simulink model "quadrotor_Euler"  (R2022b)
settings: Solver=VariableStepAuto  StartTime=0.0  StopTime=10.0  RelTol=1e-3
libraries: slpidlib x4
settings Model: SnapshotBufferSize=20  SnapshotInterval=20  Creator=user  LastModifiedBy=user

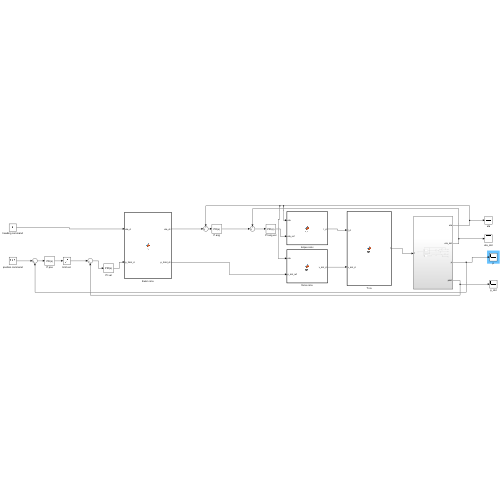
[thumbnail: Simulink's stored preview of the top-level diagram]
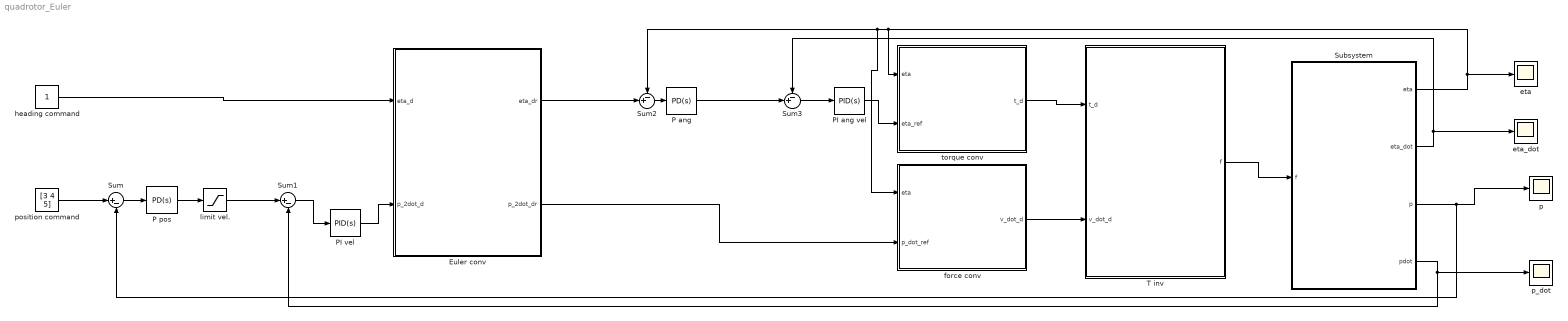
== system quadrotor_Euler ==
  Euler conv : MATLAB Function  TreatAsAtomicUnit=on
  P ang : slpidlib/PID Controller  Controller=PD  Form=Parallel  TimeDomain=Continuous-time  UseExternalTs=off  SampleTime=-1  IntegratorMethod=Forward Euler  FilterMethod=Forward Euler  ControllerParametersSource=internal  P=20  I=1  UseKiTs=off  D=0.2  N=100  UseFilter=on  TunerSelectOption=Transfer Function Based (PID Tuner App)  InitialConditionSource=internal  InitialConditionForIntegrator=0  InitialConditionForFilter=0  DifferentiatorICPrevScaledInput=0  ExternalReset=none  TrackingMode=off  Kt=1  LimitOutput=off  SatLimitsSource=internal  UpperSaturationLimit=inf  LowerSaturationLimit=-inf  LinearizeAsGain=on  AntiWindupMode=none  Kb=1  LimitIntegrator=off  UpperIntegratorSaturationLimit=inf  LowerIntegratorSaturationLimit=-inf  POutMin=[]  POutMax=[]  IOutMin=[]  IOutMax=[]  DOutMin=[]  DOutMax=[]  NOutMin=[]  NOutMax=[]  SumOutMin=[]  SumOutMax=[]  SaturationOutMin=[]  SaturationOutMax=[]  PParamMin=[]  PParamMax=[]  IParamMin=[]  IParamMax=[]  DParamMin=[]  DParamMax=[]  NParamMin=[]  NParamMax=[]  KbParamMin=[]  KbParamMax=[]  KtParamMin=[]  KtParamMax=[]  KbOutMin=[]  KbOutMax=[]  KtOutMin=[]  KtOutMax=[]  IntegratorOutMin=[]  IntegratorOutMax=[]  FilterOutMin=[]  FilterOutMax=[]  SumI1OutMin=[]  SumI1OutMax=[]  SumI2OutMin=[]  SumI2OutMax=[]  SumI3OutMin=[]  SumI3OutMax=[]  SumI4OutMin=[]  SumI4OutMax=[]  SumDOutMin=[]  SumDOutMax=[]  DifferentiatorOutMin=[]  DifferentiatorOutMax=[]  FilterDiffOutCoefMin=[]  FilterDiffOutCoefMax=[]  ReciprocalOutMin=[]  ReciprocalOutMax=[]  SumDenOutMin=[]  SumDenOutMax=[]  SumNumOutMin=[]  SumNumOutMax=[]  DivideOutMin=[]  DivideOutMax=[]  UdiffTsProdOutMin=[]  UdiffTsProdOutMax=[]  NTsProdOutMin=[]  NTsProdOutMax=[]  UintegralTsProdOutMin=[]  UintegralTsProdOutMax=[]  UngainTsProdOutMin=[]  UngainTsProdOutMax=[]  ClampingZeroOutDataTypeStr=Inherit: Inherit via back propagation  ClampingZeroOutMin=[]  ClampingZeroOutMax=[]  FilterDenConstantOutDataTypeStr=Inherit: Inherit via back propagation  FilterDenConstantOutMin=[]  FilterDenConstantOutMax=[]  PCopyOutDataTypeStr=Inherit: Inherit via back propagation  PCopyOutMin=[]  PCopyOutMax=[]  NCopyOutDataTypeStr=Inherit: Inherit via back propagation  NCopyOutMin=[]  NCopyOutMax=[]  IntegratorContinuousStateAttributes=''  IntegratorStateMustResolveToSignalObject=off  IntegratorRTWStateStorageClass=Auto  FilterContinuousStateAttributes=''  FilterStateMustResolveToSignalObject=off  FilterRTWStateStorageClass=Auto  ParallelPVariant=InternalParameters  IdealPVariant=Disabled  IVariant=Disabled  DVariant=InternalParameters  IntegratorVariant=Disabled  SatVariant=Disabled  AWVariant=Disabled  PCopyVariant=Disabled  TRVariant=Disabled  FdbkBlocksVariant=Forward  IdealPFdbkVariant=Disabled  SatFdbkVariant=Disabled  DerivativeFilterVariant=ContFilter  NVariant=InternalParameters  NCopyVariant=Disabled  FilterICVariant=InternalICsFilter  IntegratorICVariant=Disabled  ExternalResetVariant=Disabled  TRSumVariant=Passthrough  SumFdbkVariant=Disabled  SumVariant=Sum_PD  TsampFilterVariant=InternalTs  TsampNgainVariant=Passthrough  TsampIntegralVariant=Disabled_SignalSpec  ExternalSaturationOutDataTypeStr=Inherit: Same as second input
  P pos : slpidlib/PID Controller  Controller=PD  Form=Parallel  TimeDomain=Continuous-time  UseExternalTs=off  SampleTime=-1  IntegratorMethod=Forward Euler  FilterMethod=Forward Euler  ControllerParametersSource=internal  P=5  I=1  UseKiTs=off  D=0.8  N=100  UseFilter=on  TunerSelectOption=Transfer Function Based (PID Tuner App)  InitialConditionSource=internal  InitialConditionForIntegrator=0  InitialConditionForFilter=0  DifferentiatorICPrevScaledInput=0  ExternalReset=none  TrackingMode=off  Kt=1  LimitOutput=off  SatLimitsSource=internal  UpperSaturationLimit=inf  LowerSaturationLimit=-inf  LinearizeAsGain=on  AntiWindupMode=none  Kb=1  LimitIntegrator=off  UpperIntegratorSaturationLimit=inf  LowerIntegratorSaturationLimit=-inf  POutMin=[]  POutMax=[]  IOutMin=[]  IOutMax=[]  DOutMin=[]  DOutMax=[]  NOutMin=[]  NOutMax=[]  SumOutMin=[]  SumOutMax=[]  SaturationOutMin=[]  SaturationOutMax=[]  PParamMin=[]  PParamMax=[]  IParamMin=[]  IParamMax=[]  DParamMin=[]  DParamMax=[]  NParamMin=[]  NParamMax=[]  KbParamMin=[]  KbParamMax=[]  KtParamMin=[]  KtParamMax=[]  KbOutMin=[]  KbOutMax=[]  KtOutMin=[]  KtOutMax=[]  IntegratorOutMin=[]  IntegratorOutMax=[]  FilterOutMin=[]  FilterOutMax=[]  SumI1OutMin=[]  SumI1OutMax=[]  SumI2OutMin=[]  SumI2OutMax=[]  SumI3OutMin=[]  SumI3OutMax=[]  SumI4OutMin=[]  SumI4OutMax=[]  SumDOutMin=[]  SumDOutMax=[]  DifferentiatorOutMin=[]  DifferentiatorOutMax=[]  FilterDiffOutCoefMin=[]  FilterDiffOutCoefMax=[]  ReciprocalOutMin=[]  ReciprocalOutMax=[]  SumDenOutMin=[]  SumDenOutMax=[]  SumNumOutMin=[]  SumNumOutMax=[]  DivideOutMin=[]  DivideOutMax=[]  UdiffTsProdOutMin=[]  UdiffTsProdOutMax=[]  NTsProdOutMin=[]  NTsProdOutMax=[]  UintegralTsProdOutMin=[]  UintegralTsProdOutMax=[]  UngainTsProdOutMin=[]  UngainTsProdOutMax=[]  ClampingZeroOutDataTypeStr=Inherit: Inherit via back propagation  ClampingZeroOutMin=[]  ClampingZeroOutMax=[]  FilterDenConstantOutDataTypeStr=Inherit: Inherit via back propagation  FilterDenConstantOutMin=[]  FilterDenConstantOutMax=[]  PCopyOutDataTypeStr=Inherit: Inherit via back propagation  PCopyOutMin=[]  PCopyOutMax=[]  NCopyOutDataTypeStr=Inherit: Inherit via back propagation  NCopyOutMin=[]  NCopyOutMax=[]  IntegratorContinuousStateAttributes=''  IntegratorStateMustResolveToSignalObject=off  IntegratorRTWStateStorageClass=Auto  FilterContinuousStateAttributes=''  FilterStateMustResolveToSignalObject=off  FilterRTWStateStorageClass=Auto  ParallelPVariant=InternalParameters  IdealPVariant=Disabled  IVariant=Disabled  DVariant=InternalParameters  IntegratorVariant=Disabled  SatVariant=Disabled  AWVariant=Disabled  PCopyVariant=Disabled  TRVariant=Disabled  FdbkBlocksVariant=Forward  IdealPFdbkVariant=Disabled  SatFdbkVariant=Disabled  DerivativeFilterVariant=ContFilter  NVariant=InternalParameters  NCopyVariant=Disabled  FilterICVariant=InternalICsFilter  IntegratorICVariant=Disabled  ExternalResetVariant=Disabled  TRSumVariant=Passthrough  SumFdbkVariant=Disabled  SumVariant=Sum_PD  TsampFilterVariant=InternalTs  TsampNgainVariant=Passthrough  TsampIntegralVariant=Disabled_SignalSpec  ExternalSaturationOutDataTypeStr=Inherit: Same as second input
  PI ang vel : slpidlib/PID Controller  Controller=PID  Form=Parallel  TimeDomain=Continuous-time  UseExternalTs=off  SampleTime=-1  IntegratorMethod=Forward Euler  FilterMethod=Forward Euler  ControllerParametersSource=internal  P=25  I=0.0  UseKiTs=off  D=0  N=100  UseFilter=on  TunerSelectOption=Transfer Function Based (PID Tuner App)  InitialConditionSource=internal  InitialConditionForIntegrator=0  InitialConditionForFilter=0  DifferentiatorICPrevScaledInput=0  ExternalReset=none  TrackingMode=off  Kt=1  LimitOutput=off  SatLimitsSource=internal  UpperSaturationLimit=inf  LowerSaturationLimit=-inf  LinearizeAsGain=on  AntiWindupMode=none  Kb=1  LimitIntegrator=off  UpperIntegratorSaturationLimit=inf  LowerIntegratorSaturationLimit=-inf  POutMin=[]  POutMax=[]  IOutMin=[]  IOutMax=[]  DOutMin=[]  DOutMax=[]  NOutMin=[]  NOutMax=[]  SumOutMin=[]  SumOutMax=[]  SaturationOutMin=[]  SaturationOutMax=[]  PParamMin=[]  PParamMax=[]  IParamMin=[]  IParamMax=[]  DParamMin=[]  DParamMax=[]  NParamMin=[]  NParamMax=[]  KbParamMin=[]  KbParamMax=[]  KtParamMin=[]  KtParamMax=[]  KbOutMin=[]  KbOutMax=[]  KtOutMin=[]  KtOutMax=[]  IntegratorOutMin=[]  IntegratorOutMax=[]  FilterOutMin=[]  FilterOutMax=[]  SumI1OutMin=[]  SumI1OutMax=[]  SumI2OutMin=[]  SumI2OutMax=[]  SumI3OutMin=[]  SumI3OutMax=[]  SumI4OutMin=[]  SumI4OutMax=[]  SumDOutMin=[]  SumDOutMax=[]  DifferentiatorOutMin=[]  DifferentiatorOutMax=[]  FilterDiffOutCoefMin=[]  FilterDiffOutCoefMax=[]  ReciprocalOutMin=[]  ReciprocalOutMax=[]  SumDenOutMin=[]  SumDenOutMax=[]  SumNumOutMin=[]  SumNumOutMax=[]  DivideOutMin=[]  DivideOutMax=[]  UdiffTsProdOutMin=[]  UdiffTsProdOutMax=[]  NTsProdOutMin=[]  NTsProdOutMax=[]  UintegralTsProdOutMin=[]  UintegralTsProdOutMax=[]  UngainTsProdOutMin=[]  UngainTsProdOutMax=[]  ClampingZeroOutDataTypeStr=Inherit: Inherit via back propagation  ClampingZeroOutMin=[]  ClampingZeroOutMax=[]  FilterDenConstantOutDataTypeStr=Inherit: Inherit via back propagation  FilterDenConstantOutMin=[]  FilterDenConstantOutMax=[]  PCopyOutDataTypeStr=Inherit: Inherit via back propagation  PCopyOutMin=[]  PCopyOutMax=[]  NCopyOutDataTypeStr=Inherit: Inherit via back propagation  NCopyOutMin=[]  NCopyOutMax=[]  IntegratorContinuousStateAttributes=''  IntegratorStateMustResolveToSignalObject=off  IntegratorRTWStateStorageClass=Auto  FilterContinuousStateAttributes=''  FilterStateMustResolveToSignalObject=off  FilterRTWStateStorageClass=Auto  ParallelPVariant=InternalParameters  IdealPVariant=Disabled  IVariant=InternalParameters  DVariant=InternalParameters  IntegratorVariant=Continuous  SatVariant=Disabled  AWVariant=Passthrough  PCopyVariant=Disabled  TRVariant=Disabled  FdbkBlocksVariant=Forward  IdealPFdbkVariant=Disabled  SatFdbkVariant=Disabled  DerivativeFilterVariant=ContFilter  NVariant=InternalParameters  NCopyVariant=Disabled  FilterICVariant=InternalICsFilter  IntegratorICVariant=InternalICs  ExternalResetVariant=Disabled  TRSumVariant=Passthrough  SumFdbkVariant=Disabled  SumVariant=Sum_PID  TsampFilterVariant=InternalTs  TsampNgainVariant=Passthrough  TsampIntegralVariant=Passthrough  ExternalSaturationOutDataTypeStr=Inherit: Same as second input
  PI vel : slpidlib/PID Controller  Controller=PID  Form=Parallel  TimeDomain=Continuous-time  UseExternalTs=off  SampleTime=-1  IntegratorMethod=Forward Euler  FilterMethod=Forward Euler  ControllerParametersSource=internal  P=18  I=0.2  UseKiTs=off  D=1  N=100  UseFilter=on  TunerSelectOption=Transfer Function Based (PID Tuner App)  InitialConditionSource=internal  InitialConditionForIntegrator=0  InitialConditionForFilter=0  DifferentiatorICPrevScaledInput=0  ExternalReset=none  TrackingMode=off  Kt=1  LimitOutput=off  SatLimitsSource=internal  UpperSaturationLimit=inf  LowerSaturationLimit=-inf  LinearizeAsGain=on  AntiWindupMode=none  Kb=1  LimitIntegrator=off  UpperIntegratorSaturationLimit=inf  LowerIntegratorSaturationLimit=-inf  POutMin=[]  POutMax=[]  IOutMin=[]  IOutMax=[]  DOutMin=[]  DOutMax=[]  NOutMin=[]  NOutMax=[]  SumOutMin=[]  SumOutMax=[]  SaturationOutMin=[]  SaturationOutMax=[]  PParamMin=[]  PParamMax=[]  IParamMin=[]  IParamMax=[]  DParamMin=[]  DParamMax=[]  NParamMin=[]  NParamMax=[]  KbParamMin=[]  KbParamMax=[]  KtParamMin=[]  KtParamMax=[]  KbOutMin=[]  KbOutMax=[]  KtOutMin=[]  KtOutMax=[]  IntegratorOutMin=[]  IntegratorOutMax=[]  FilterOutMin=[]  FilterOutMax=[]  SumI1OutMin=[]  SumI1OutMax=[]  SumI2OutMin=[]  SumI2OutMax=[]  SumI3OutMin=[]  SumI3OutMax=[]  SumI4OutMin=[]  SumI4OutMax=[]  SumDOutMin=[]  SumDOutMax=[]  DifferentiatorOutMin=[]  DifferentiatorOutMax=[]  FilterDiffOutCoefMin=[]  FilterDiffOutCoefMax=[]  ReciprocalOutMin=[]  ReciprocalOutMax=[]  SumDenOutMin=[]  SumDenOutMax=[]  SumNumOutMin=[]  SumNumOutMax=[]  DivideOutMin=[]  DivideOutMax=[]  UdiffTsProdOutMin=[]  UdiffTsProdOutMax=[]  NTsProdOutMin=[]  NTsProdOutMax=[]  UintegralTsProdOutMin=[]  UintegralTsProdOutMax=[]  UngainTsProdOutMin=[]  UngainTsProdOutMax=[]  ClampingZeroOutDataTypeStr=Inherit: Inherit via back propagation  ClampingZeroOutMin=[]  ClampingZeroOutMax=[]  FilterDenConstantOutDataTypeStr=Inherit: Inherit via back propagation  FilterDenConstantOutMin=[]  FilterDenConstantOutMax=[]  PCopyOutDataTypeStr=Inherit: Inherit via back propagation  PCopyOutMin=[]  PCopyOutMax=[]  NCopyOutDataTypeStr=Inherit: Inherit via back propagation  NCopyOutMin=[]  NCopyOutMax=[]  IntegratorContinuousStateAttributes=''  IntegratorStateMustResolveToSignalObject=off  IntegratorRTWStateStorageClass=Auto  FilterContinuousStateAttributes=''  FilterStateMustResolveToSignalObject=off  FilterRTWStateStorageClass=Auto  ParallelPVariant=InternalParameters  IdealPVariant=Disabled  IVariant=InternalParameters  DVariant=InternalParameters  IntegratorVariant=Continuous  SatVariant=Disabled  AWVariant=Passthrough  PCopyVariant=Disabled  TRVariant=Disabled  FdbkBlocksVariant=Forward  IdealPFdbkVariant=Disabled  SatFdbkVariant=Disabled  DerivativeFilterVariant=ContFilter  NVariant=InternalParameters  NCopyVariant=Disabled  FilterICVariant=InternalICsFilter  IntegratorICVariant=InternalICs  ExternalResetVariant=Disabled  TRSumVariant=Passthrough  SumFdbkVariant=Disabled  SumVariant=Sum_PID  TsampFilterVariant=InternalTs  TsampNgainVariant=Passthrough  TsampIntegralVariant=Passthrough  ExternalSaturationOutDataTypeStr=Inherit: Same as second input
  Subsystem : Subsystem
  Sum : Sum  Inputs=|+-
  Sum1 : Sum  Inputs=|+-
  Sum2 : Sum  Inputs=-+|
  Sum3 : Sum  Inputs=-+|
  T inv : MATLAB Function  TreatAsAtomicUnit=on
  eta : Scope
  eta_dot : Scope
  force conv : MATLAB Function  TreatAsAtomicUnit=on
  heading command : Constant
  limit vel. : Saturate  UpperLimit=5  LowerLimit=-1
  p : Scope
  p_dot : Scope
  position command : Constant  Value=[3 4 5]  VectorParams1D=off
  torque conv : MATLAB Function  TreatAsAtomicUnit=on
  wires:
  Sum/1 -> P pos/1
  P pos/1 -> limit vel./1
  Sum1/1 -> PI vel/1
  position command/1 -> Sum/1
  heading command/1 -> Euler conv/1(eta_d)
  PI vel/1 -> Euler conv/2(p_2dot_d)
  Sum2/1 -> P ang/1
  Sum3/1 -> PI ang vel/1
  PI ang vel/1 -> torque conv/2(eta_ref)
  force conv/1(v_dot_d) -> T inv/2(v_dot_d)
  torque conv/1(t_d) -> T inv/1(t_d)
  Subsystem/4(pdot) -> p_dot/1, Sum1/2
  Subsystem/3(p) -> p/1, Sum/2
  Subsystem/1(eta) -> eta/1, torque conv/1(eta), force conv/1(eta), Sum2/1
  Subsystem/2(eta_dot) -> Sum3/1, eta_dot/1
  T inv/1(f) -> Subsystem/1(f)
  P ang/1 -> Sum3/2
  Euler conv/2(p_2dot_dr) -> force conv/2(p_dot_ref)
  Euler conv/1(eta_dr) -> Sum2/2
  limit vel./1 -> Sum1/1

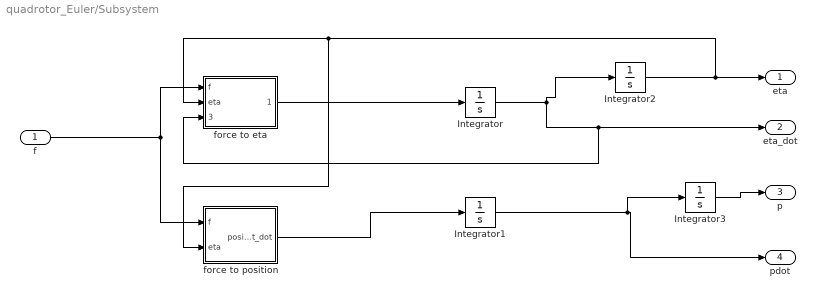
== system quadrotor_Euler/Subsystem ==
  f : Inport
  Integrator{,1..3} (4 alike) : Integrator  InitialCondition=[0 0 0]
  force to eta : MATLAB Function  TreatAsAtomicUnit=on
  force to position : MATLAB Function  TreatAsAtomicUnit=on
  eta : Outport
  eta_dot : Outport  Port=2
  p : Outport  Port=3
  pdot : Outport  Port=4
  wires:
  Integrator/1 -> Integrator2/1, force to eta/3(eta_dot), eta_dot/1
  Integrator2/1 -> force to position/2(eta), force to eta/2(eta), eta/1
  Integrator1/1 -> Integrator3/1, pdot/1
  Integrator3/1 -> p/1
  f/1 -> force to eta/1(f), force to position/1(f)
  force to eta/1(eta_dot_dot) -> Integrator/1
  force to position/1(position_dot_dot) -> Integrator1/1

== matlab function quadrotor_Euler/torque conv ==
  data: eta input size=[1,3]; t_d output size=[1,3]; eta_ref input size=[1,3]
function t_d = fcn(eta,eta_ref)

%x에 - 붙혀버림
%(원래 식:)
C = [1,0,-sin(eta(2));0,cos(eta(1)),sin(eta(1))*cos(eta(2));0,-sin(eta(1)),cos(eta(1))*cos(eta(2))];
%C = [-1,0,sin(eta(2));0,cos(eta(1)),sin(eta(1))*cos(eta(2));0,-sin(eta(1)),cos(eta(1))*cos(eta(2))];
t_d = transpose(C*transpose(eta_ref));

end

== matlab function quadrotor_Euler/Euler conv ==
  data: eta_d input size=1; eta_dr output size=[1,3]; p_2dot_d input size=[1,3]; p_2dot_dr output size=[1,3]
function [eta_dr,p_2dot_dr] = fcn(eta_d,p_2dot_d)
eta_dr=[0,0,0];
g_z = -9.81;
p_2dot_dr=[0,0,p_2dot_d(3)+9.81];
eta_dr(1)= (p_2dot_d(1)*sin(eta_d)-p_2dot_d(2)*cos(eta_d))/sqrt(p_2dot_d(1)^2+p_2dot_d(2)^2+(p_2dot_d(3)-g_z)^2);
eta_dr(2)= (p_2dot_d(1)*cos(eta_d)+p_2dot_d(2)*sin(eta_d))/(p_2dot_d(3)-g_z);
eta_dr(3)=eta_d;

end

== matlab function quadrotor_Euler/force conv ==
  data: eta input; v_dot_d output size=[1,3]; p_dot_ref input
function v_dot_d = fcn(eta,p_dot_ref)
R=[cos(eta(2))*cos(eta(3)),sin(eta(1))*sin(eta(2))*cos(eta(3))-cos(eta(1))*sin(eta(3)),cos(eta(1))*sin(eta(2))*cos(eta(3))+sin(eta(1))*sin(eta(3));
    cos(eta(2))*sin(eta(3)),sin(eta(1))*sin(eta(2))*sin(eta(3))+cos(eta(1))*cos(eta(3)),cos(eta(1))*sin(eta(2))*sin(eta(3))-sin(eta(1))*cos(eta(3));
    -sin(eta(2)),sin(eta(1))*cos(eta(2)),cos(eta(1))*cos(eta(2))];
v_dot_d=transpose(R\transpose(p_dot_ref));
end

== matlab function quadrotor_Euler/T inv ==
  data: t_d input; f output size=[1,4]; v_dot_d input
function f = fcn(t_d,v_dot_d)
u=[v_dot_d(3),t_d(1),t_d(2),t_d(3)];
m=1;
l=1;
r=0.2;
T=[1/m,1/m,1/m,1/m ; 0,-l,0,l ; -l,0,l,0 ; r,-r,r,-r];
f=transpose(T\transpose(u));

end

== matlab function quadrotor_Euler/Subsystem/force to eta ==
  data: f input size=[1,4]; eta_dot_dot output size=[1,3]; eta input size=[1,3]; eta_dot input size=[1,3]
function eta_dot_dot = fcn(f,eta,eta_dot)
%C,C_dot [3,3]
C = [1,0,-sin(eta(2)) ; 0,cos(eta(1)),sin(eta(1))*cos(eta(2)) ; 0,-sin(eta(1)),cos(eta(1))*cos(eta(2))];
C_dot = [0,0,-eta_dot(2)*cos(eta(2));
    0,-eta_dot(1)*sin(eta(1)),eta_dot(1)*cos(eta(1))*cos(eta(2))-eta_dot(2)*sin(eta(1))*sin(eta(2));
    0,-eta_dot(1)*cos(eta(1)),-eta_dot(1)*sin(eta(1))*cos(eta(2))-eta_dot(2)*cos(eta(1))*sin(eta(2))];
l=1;
% Q,Omega_G [3,1]
Q=[l*(f(4)-f(2));l*(f(3)-f(1));f(1)-f(2)+f(3)-f(4)];
Omega_G=[0;0;sqrt(abs(f(1)))-sqrt(abs(f(2)))+sqrt(abs(f(3)))-sqrt(abs(f(4)))];
%eta_dot_dot은 [1,3]으로 나갈 것.
%cross([3,1],[3,1])
eta_dot_dot=transpose(C\(Q-C_dot*transpose(eta_dot)-cross(C*transpose(eta_dot),(C*transpose(eta_dot)+Omega_G))));
end

== matlab function quadrotor_Euler/Subsystem/force to position ==
  data: f input size=[1,4]; position_dot_dot output size=[1,3]; eta input size=[1,3]
function position_dot_dot = fcn(f,eta)
g=[0;0;-9.8];
F=[0;0;f(1)+f(2)+f(3)+f(4)];
m=1;
M=[1/m,0,0 ; 0,1/m,0 ; 0,0,1/m];

R=[cos(eta(2))*cos(eta(3)),sin(eta(1))*sin(eta(2))*cos(eta(3))-cos(eta(1))*sin(eta(3)),cos(eta(1))*sin(eta(2))*cos(eta(3))+sin(eta(1))*sin(eta(3));
    cos(eta(2))*sin(eta(3)),sin(eta(1))*sin(eta(2))*sin(eta(3))+cos(eta(1))*cos(eta(3)),cos(eta(1))*sin(eta(2))*sin(eta(3))-sin(eta(1))*cos(eta(3));
    -sin(eta(2)),sin(eta(1))*cos(eta(2)),cos(eta(1))*cos(eta(2))];

position_dot_dot=transpose(g+M*R*F);

end
